simulink model "ers"  (R2024a)
settings: Solver=VariableStepAuto  StartTime=0.0  StopTime=10.0  RelTol=1e-3
settings Model: Creator=DELL  LastModifiedBy=DELL

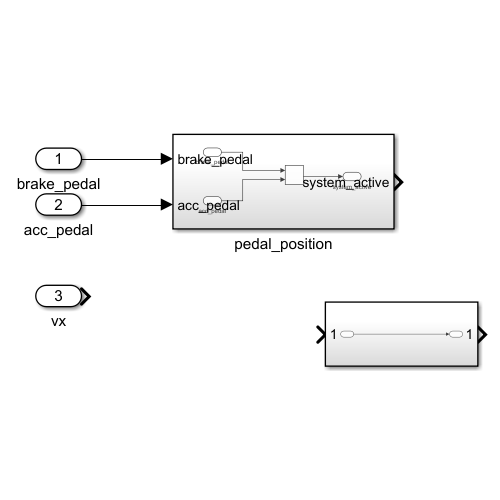
[thumbnail: Simulink's stored preview of the top-level diagram]
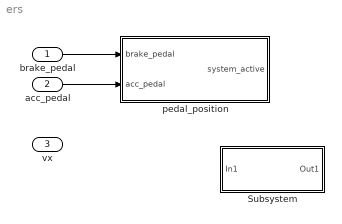
== system ers ==
  brake_pedal : Inport
  acc_pedal : Inport  Port=2
  vx : Inport  Port=3
  Subsystem : Subsystem
  pedal_position : Subsystem
  wires:
  brake_pedal/1 -> pedal_position/1(brake_pedal)
  acc_pedal/1 -> pedal_position/2(acc_pedal)

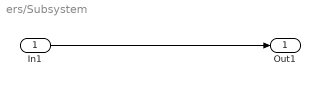
== system ers/Subsystem ==
  In1 : Inport
  Out1 : Outport
  wires:
  In1/1 -> Out1/1

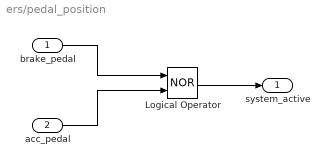
== system ers/pedal_position ==
  brake_pedal : Inport
  acc_pedal : Inport  Port=2
  Logical Operator : Logic  Operator=NOR  AllPortsSameDT=off  OutDataTypeStr=boolean
  system_active : Outport
  wires:
  brake_pedal/1 -> Logical Operator/1
  acc_pedal/1 -> Logical Operator/2
  Logical Operator/1 -> system_active/1
